simulink model "PendulumFeedback"  (R2019b)
settings: Solver=VariableStepAuto  StartTime=0.0  StopTime=10.0  RelTol=1e-3
settings Model: Creator=aarij  LastModifiedBy=aarij

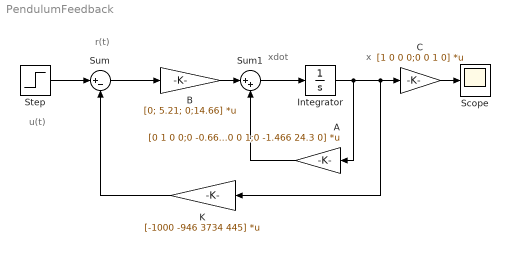
== system PendulumFeedback ==
  note: u(t)
  note: x
  note: xdot
  note: r(t)
  A : Gain  Gain=[0 1 0 0;0 -0.661 1.265 0; 0 0 0 1;0 -1.466 24.3 0]  Multiplication=Matrix(K*u)
  B : Gain  Gain=[0; 5.21; 0;14.66]  Multiplication=Matrix(K*u) (u vector)
  C : Gain  Gain=[1 0 0 0;0 0 1 0]  Multiplication=Matrix(K*u)
  Integrator : Integrator
  K : Gain  Gain=[-1000 -946 3734 445]  Multiplication=Matrix(K*u)
  Scope : Scope
  Step : Step  Time=0  SampleTime=0
  Sum : Sum  Inputs=|+-
  Sum1 : Sum  Inputs=|++
  wires:
  Step/1 -> Sum/1
  B/1 -> Sum1/1
  Sum/1 -> B/1
  Integrator/1 -> A/1, K/1, C/1
  Sum1/1 -> Integrator/1
  A/1 -> Sum1/2
  K/1 -> Sum/2
  C/1 -> Scope/1
